simulink model "position"  (R2018b)
settings: Solver=VariableStepAuto  StartTime=0.0  StopTime=10  RelTol=1e-3
values from neighbouring files (symbols this model uses):
  A = [0,1,0,0;-ks/Il,-cl/Il,ks/Il,0;0,0,0,1;ks/Im,0,-ks/Im,-cm/Im]    [base_mix.m]    (also in optimal_control.m)
  B = [0,0;0,1/Il;0,0;K/Im,0]    [base_mix.m]    (also in optimal_control.m)
  C = [0,0,1,0;1,0,0,0;-ks,0,ks,0]    [base_mix.m]    (also in optimal_control.m)
  D = zeros(3,2)    [base_mix.m]    (also in optimal_control.m)
  G = G(4)    [base_mix.m]    (also in optimal_control.m)
  Kf = acker(A,B(:,1),Target_Pole)    [base_mix.m]    (also in optimal_control.m = lqr(A,B(:,1),Q,R))
libraries: cstblocks x1
settings Model: Creator=78224  LastModifiedBy=78224

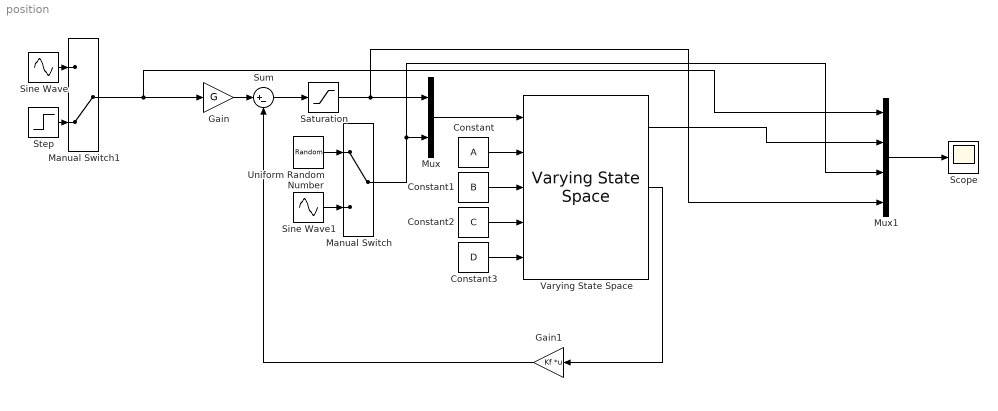
== system position ==
  Constant : Constant  Value=A  VectorParams1D=off
  Constant1 : Constant  Value=B  VectorParams1D=off
  Constant2 : Constant  Value=C  VectorParams1D=off
  Constant3 : Constant  Value=D  VectorParams1D=off
  Gain : Gain  Gain=G
  Gain1 : Gain  Gain=Kf  Multiplication=Matrix(K*u)
  Manual Switch : ManualSwitch
  Manual Switch1 : ManualSwitch  CurrentSetting=0
  Mux : Mux  Inputs=2
  Mux1 : Mux
  Saturation : Saturate  UpperLimit=3.12  LowerLimit=-3.12
  Scope : Scope
  Sine Wave : Sin  Amplitude=30  Frequency=2*pi*0.2  SampleTime=0
  Sine Wave1 : Sin  Amplitude=0  Frequency=2*pi*0.2  SampleTime=0
  Step : Step  After=30  SampleTime=0
  Sum : Sum  Inputs=|+-
  Uniform Random Number : UniformRandomNumber  Minimum=-5  Maximum=5  SampleTime=0.2
  Varying State Space : cstblocks/Linear Parameter Varying/Varying State Space  x0=0  xNames=''  OutputX=on  OutputDX=on
      settings: SourceProductName=Control System Toolbox
  wires:
  Constant/1 -> Varying State Space/2
  Constant1/1 -> Varying State Space/3
  Constant2/1 -> Varying State Space/4
  Constant3/1 -> Varying State Space/5
  Mux1/1 -> Scope/1
  Manual Switch1/1 -> Gain/1, Mux1/1
  Mux/1 -> Varying State Space/1
  Manual Switch/1 -> Mux1/3, Mux/2
  Varying State Space/2 -> Gain1/1
  Gain/1 -> Sum/1
  Sum/1 -> Saturation/1
  Gain1/1 -> Sum/2
  Varying State Space/1 -> Mux1/2
  Uniform Random Number/1 -> Manual Switch/1
  Sine Wave1/1 -> Manual Switch/2
  Step/1 -> Manual Switch1/2
  Sine Wave/1 -> Manual Switch1/1
  Saturation/1 -> Mux1/4, Mux/1
